simulink model "blockdemo"  (Simulink 6.3)
settings: Solver=ode45  StartTime=0.0  StopTime=10.0  RelTol=1e-3
InitFcn:
  | %% DSPBuilder Start
  | alt_dspbuilder_update_model(bdroot)
  | %% DSPBuilder End
libraries: allblocks_alteradspbuilder2 x7
settings Model: Creator=cpurcell  LastModifiedBy=delphick
settings DebuggingCC: MultiTaskDSMMsg=error

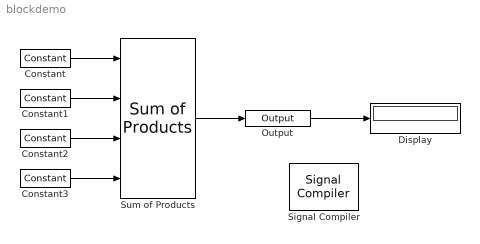
== system blockdemo ==
  Constant : allblocks_alteradspbuilder2/Constant  mask_cst=5  BusType=Signed Integer  bwl=4  bwr=0  SpecifyClock=off
  Constant1 : allblocks_alteradspbuilder2/Constant  mask_cst=7  BusType=Signed Integer  bwl=4  bwr=0  SpecifyClock=off
  Constant2 : allblocks_alteradspbuilder2/Constant  mask_cst=-5  BusType=Signed Integer  bwl=4  bwr=0  SpecifyClock=off
  Constant3 : allblocks_alteradspbuilder2/Constant  mask_cst=-8  BusType=Signed Integer  bwl=4  bwr=0  SpecifyClock=off
  Display : Display
  Output : allblocks_alteradspbuilder2/Output  iofile=C:\workspace_clean\Documentation\DesignExamples\Tutorials\UnitBlocks\Arithmetic\SumOfProducts\tb_blockdemo\blockdemo_Output.capture  BusType=Inferred  bwl=8  bwr=0  PORTTYPE=Output
  Signal Compiler : allblocks_alteradspbuilder2/Signal Compiler  DeviceFamily=Stratix IV  DeviceName=AUTO  EnableSignalTap=off  SignalTapDepth=128  UseBoardBlock=off  StpUseDefaultClock=on  StpClock=clock
  Sum of Products : allblocks_alteradspbuilder2/Sum of Products  BusType=Signed Integer  InputBwl=4  InputBwr=0  number_of_coefficients=4  CoefBwl=8  CoefBwr=0  coefficients=[4 64 -4 -64]  pipeline=0  full_resolution=on  OutputBwl=8  OutputBwr=0  TruncateLsb=0  implementation=Auto  use_ena=off  use_aclr=off
  wires:
  Constant/1 -> Sum of Products/1
  Constant1/1 -> Sum of Products/2
  Constant2/1 -> Sum of Products/3
  Constant3/1 -> Sum of Products/4
  Sum of Products/1 -> Output/1
  Output/1 -> Display/1
